simulink model "Simulink_ABS_Braking_Vehicle_Dynamics"  (R2024b)
settings: Solver=VariableStepAuto  StartTime=0.0  StopTime=10.0  RelTol=1e-3
values from neighbouring files (symbols this model uses):
  delta = 5 * pi/180    (= 0.0872664625997)    [ABS_MAtlab_Script_Automation.m]
  I_w = 1.12    [ABS_MAtlab_Script_Automation.m]
  lambda_bp = (0:0.05:1)'    [ABS_MAtlab_Script_Automation.m]
  m = 1400    [ABS_MAtlab_Script_Automation.m]
  mu_dry = ([0.00  0.40  0.80  0.97  1.00  0.98  0.96  0.94  0.92  0.90 0.88  0.85  0.83  0.81  0.79  0.77  0.75  0.73  0.72  0.71  0.70 ])'    [ABS_MAtlab_Script_Automation.m]
  mu_ice = ([0.00  0.05  0.10  0.12  0.13  0.14  0.14  0.14  0.14  0.14  0.14  0.14  0.14  0.14  0.14  0.14  0.14  0.14  0.14  0.14  0.14 ])'    [ABS_MAtlab_Script_Automation.m]
  mu_wet = ([0.00  0.25  0.45  0.55  0.60  0.62  0.61  0.60  0.59  0.58 0.57  0.56  0.55  0.54  0.53  0.52  0.50  0.48  0.46  0.44  0.42 ])'    [ABS_MAtlab_Script_Automation.m]
  r = 0.33    [ABS_MAtlab_Script_Automation.m]
  T_brake = 2000    [ABS_MAtlab_Script_Automation.m]
  v0 = 100/3.6    (= 27.7777777778)    [ABS_MAtlab_Script_Automation.m]
  w0 = v0/r    (= 84.1750841751)    [ABS_MAtlab_Script_Automation.m]
libraries: simulink x8, slpidlib x4
(part 1 of 2)
settings Model: Creator=mohammed omrez khan  LastModifiedBy=mohammed omrez khan

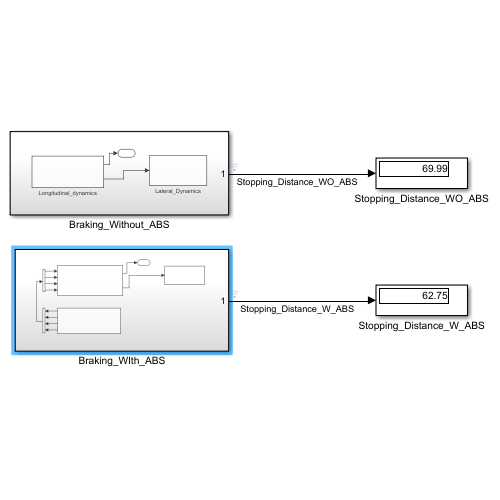
[thumbnail: Simulink's stored preview of the top-level diagram]
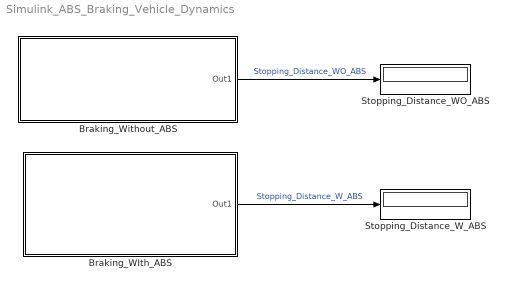
== system Simulink_ABS_Braking_Vehicle_Dynamics ==
  Braking_WIth_ABS : Subsystem
  Braking_Without_ABS : Subsystem
  Stopping_Distance_WO_ABS : Display
  Stopping_Distance_W_ABS : Display
  wires:
  Braking_Without_ABS/1(Out1) -> Stopping_Distance_WO_ABS/1  "Stopping_Distance_WO_ABS"
  Braking_WIth_ABS/1(Out1) -> Stopping_Distance_W_ABS/1  "Stopping_Distance_W_ABS"

== system Simulink_ABS_Braking_Vehicle_Dynamics/Braking_WIth_ABS ==
  Demux : Demux
  Lateral_Dynamics_ABS : Subsystem
  Longitudinal_Dynamics_ABS : Subsystem
  Mux : Mux
  Usage_ECS_Monitoring : Subsystem
      settings: PortSchema="{\"entries\":[{\"content\":{\"sides\":[{\"content\":{\"connectorIds\":[\"Out1\",\"Out2\",\"Out3\",\"Out4\"]},\"type\":\"ConnectorPlacement.EquallySpacedRectSide\",\"uuid\":\"f2e56514-8109-4cf8-b4cd-59c3b61fcd4b\"},{\"content\":{\"side\":\"RIGHT\"},\"type\":\"ConnectorPlacement.EquallySpacedRectSide\",\"uuid\":\"6eb04186-cc68-428c-910d-d8e45f75c5ef\"},{\"content\":{\"side\":\"TOP\"},\"type\":\"ConnectorPlacement.EquallySpacedRectSide\",\"uuid\":\"72babd61-98dc-4993-babf-b2ef769bf457\"}]},\"type\":\"ConnectorPlacement.EquallySpacedConnector\",\"uuid\":\"fac04954-b134-470d-b15d-7da1141ea9e2\"}],\"packageUris\":[\"http://schema.mathworks.com/mf0/Connector/R2020b\"],\"version\":\"1.0\"}"
  Out1 : Outport
  wires:
  Longitudinal_Dynamics_ABS/1(Out1) -> Out1/1
  Longitudinal_Dynamics_ABS/2(V_x) -> Lateral_Dynamics_ABS/1(V_x)
  Usage_ECS_Monitoring/1(Out1) -> Mux/1
  Usage_ECS_Monitoring/2(Out2) -> Mux/2
  Usage_ECS_Monitoring/3(Out3) -> Mux/3
  Usage_ECS_Monitoring/4(Out4) -> Mux/4
  Mux/1 -> Demux/1
  Demux/1 -> Longitudinal_Dynamics_ABS/1(In1)
  Demux/2 -> Longitudinal_Dynamics_ABS/2(In2)
  Demux/3 -> Longitudinal_Dynamics_ABS/3(In3)
  Demux/4 -> Longitudinal_Dynamics_ABS/4(In4)

== system Simulink_ABS_Braking_Vehicle_Dynamics/Braking_Without_ABS ==
  Lateral_Dynamics : Subsystem
  Longitudinal_dynamics : Subsystem
  Out1 : Outport
  wires:
  Longitudinal_dynamics/1(Out1) -> Out1/1
  Longitudinal_dynamics/2(V_x) -> Lateral_Dynamics/1(V_x)

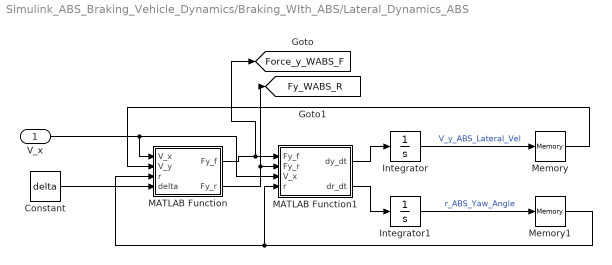
== system Simulink_ABS_Braking_Vehicle_Dynamics/Braking_WIth_ABS/Lateral_Dynamics_ABS ==
  V_x : Inport
  Constant : Constant  Value=delta
  Integrator : Integrator
  Integrator1 : Integrator
  MATLAB Function : MATLAB Function  TreatAsAtomicUnit=on
  MATLAB Function1 : MATLAB Function  TreatAsAtomicUnit=on
  Memory : Memory
  Memory1 : Memory
  tag scope: Force_y_WABS_F=global, Fy_WABS_R=global
  wires:
  MATLAB Function1/1(dy_dt) -> Integrator/1
  Constant/1 -> MATLAB Function/4(delta)
  MATLAB Function1/2(dr_dt) -> Integrator1/1
  MATLAB Function/1(Fy_f) -> [Force_y_WABS_F], MATLAB Function1/1(Fy_f)
  V_x/1 -> MATLAB Function/1(V_x), MATLAB Function1/3(V_x)
  Integrator/1 -> Memory/1  "V_y_ABS_Lateral_Vel"
  Memory/1 -> MATLAB Function/2(V_y)
  Integrator1/1 -> Memory1/1  "r_ABS_Yaw_Angle"
  Memory1/1 -> MATLAB Function/3(r), MATLAB Function1/4(r)
  MATLAB Function/2(Fy_r) -> [Fy_WABS_R], MATLAB Function1/2(Fy_r)

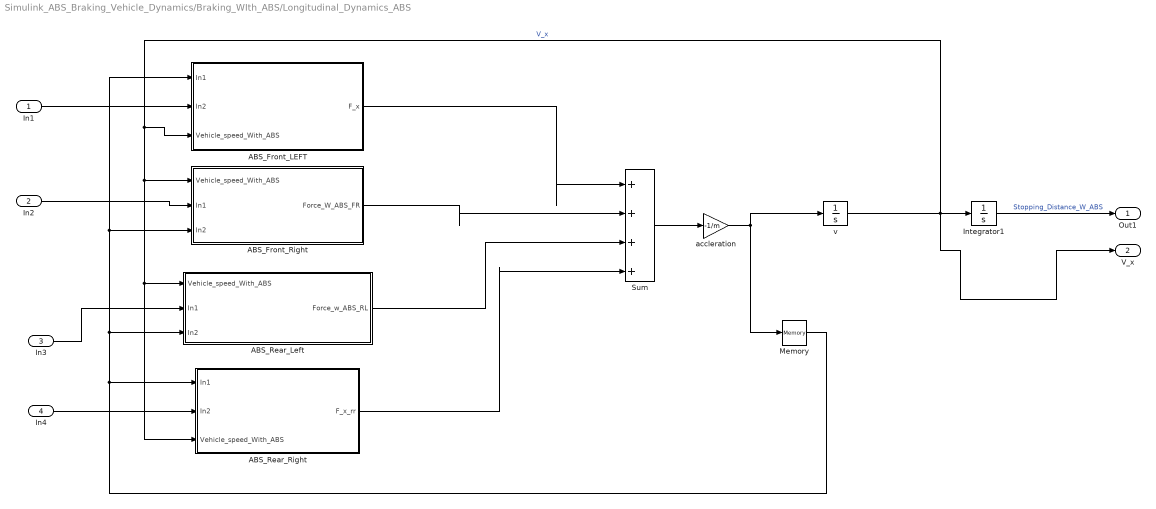
== system Simulink_ABS_Braking_Vehicle_Dynamics/Braking_WIth_ABS/Longitudinal_Dynamics_ABS ==
  In1 : Inport
  In2 : Inport  Port=2
  In3 : Inport  Port=3
  In4 : Inport  Port=4
  ABS_Front_LEFT : Subsystem
  ABS_Front_Right : Subsystem
  ABS_Rear_Left : Subsystem
  ABS_Rear_Right : Subsystem
  Integrator1 : Integrator
  Memory : Memory
  Sum : Sum  Inputs=|++++
  accleration : Gain  Gain=-1/m
  v : Integrator  InitialCondition=v0  LimitOutput=on  LowerSaturationLimit=0
  Out1 : Outport
  V_x : Outport  Port=2
  wires:
  Sum/1 -> accleration/1
  Memory/1 -> ABS_Front_LEFT/1(In1), ABS_Front_Right/3(In2), ABS_Rear_Left/3(In2), ABS_Rear_Right/1(In1)
  v/1 -> V_x/1, ABS_Rear_Right/3(Vehicle_speed_With_ABS), ABS_Rear_Left/1(Vehicle_speed_With_ABS), ABS_Front_Right/1(Vehicle_speed_With_ABS), ABS_Front_LEFT/3(Vehicle_speed_With_ABS), Integrator1/1  "V_x"
  accleration/1 -> v/1, Memory/1
  ABS_Rear_Right/1(F_x_rr) -> Sum/4
  ABS_Rear_Left/1(Force_w_ABS_RL) -> Sum/3
  ABS_Front_Right/1(Force_W_ABS_FR) -> Sum/2
  ABS_Front_LEFT/1(F_x) -> Sum/1
  Integrator1/1 -> Out1/1  "Stopping_Distance_W_ABS"
  In1/1 -> ABS_Front_LEFT/2(In2)
  In2/1 -> ABS_Front_Right/2(In1)
  In3/1 -> ABS_Rear_Left/2(In1)
  In4/1 -> ABS_Rear_Right/2(In2)

== system Simulink_ABS_Braking_Vehicle_Dynamics/Braking_WIth_ABS/Usage_ECS_Monitoring ==
  Front_Left Wheel : Subsystem
  Front_Right_Wheel : Subsystem
  Rear_Left_Wheel : Subsystem
  Rear_Right_Wheel : Subsystem
  Out1 : Outport
  Out2 : Outport  Port=2
  Out3 : Outport  Port=3
  Out4 : Outport  Port=4
  wires:
  Front_Left Wheel/1(Out1) -> Out1/1
  Front_Right_Wheel/1(Out1) -> Out2/1
  Rear_Left_Wheel/1(Out3) -> Out3/1
  Rear_Right_Wheel/1(Out3) -> Out4/1

== system Simulink_ABS_Braking_Vehicle_Dynamics/Braking_Without_ABS/Lateral_Dynamics ==
  V_x : Inport
  Constant : Constant  Value=delta
  Integrator : Integrator
  Integrator1 : Integrator
  MATLAB Function : MATLAB Function  TreatAsAtomicUnit=on
  MATLAB Function1 : MATLAB Function  TreatAsAtomicUnit=on
  Memory : Memory
  Memory1 : Memory
  wires:
  MATLAB Function/2(Fy_r) -> MATLAB Function1/2(Fy_r)
  MATLAB Function1/1(dy_dt) -> Integrator/1
  Constant/1 -> MATLAB Function/4(delta)
  MATLAB Function1/2(dr_dt) -> Integrator1/1
  MATLAB Function/1(Fy_f) -> MATLAB Function1/1(Fy_f)
  V_x/1 -> MATLAB Function/1(V_x), MATLAB Function1/3(V_x)
  Integrator/1 -> Memory/1  "V_y_velocity in Lateral"
  Memory/1 -> MATLAB Function/2(V_y)
  Integrator1/1 -> Memory1/1  "r_Yaw_Angle"
  Memory1/1 -> MATLAB Function1/4(r), MATLAB Function/3(r)

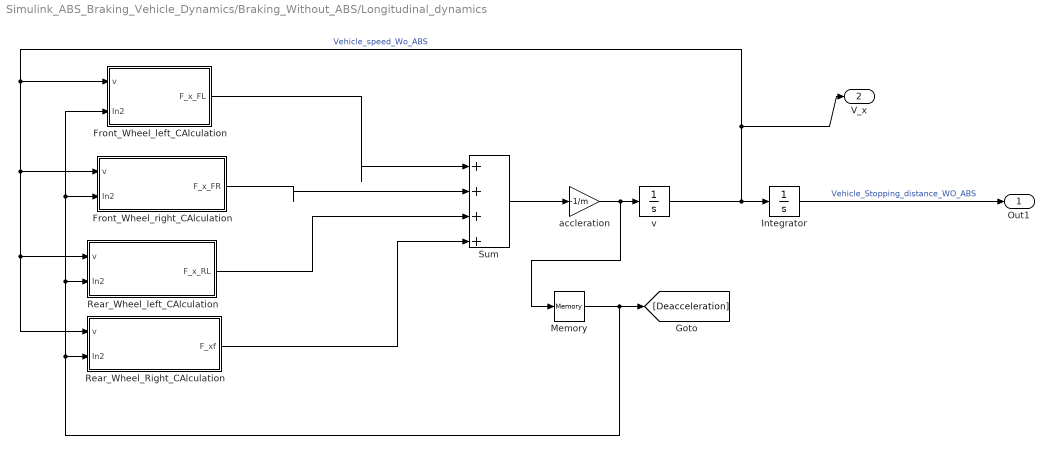
== system Simulink_ABS_Braking_Vehicle_Dynamics/Braking_Without_ABS/Longitudinal_dynamics ==
  Front_Wheel_left_CAlculation : Subsystem
  Front_Wheel_right_CAlculation : Subsystem
  Integrator : Integrator
  Memory : Memory
  Rear_Wheel_Right_CAlculation : Subsystem
  Rear_Wheel_left_CAlculation : Subsystem
  Sum : Sum  Inputs=|++++
  accleration : Gain  Gain=-1/m
  v : Integrator  InitialCondition=v0  LimitOutput=on  LowerSaturationLimit=0
  Out1 : Outport
  V_x : Outport  Port=2
  wires:
  Memory/1 -> Front_Wheel_left_CAlculation/2(In2), Front_Wheel_right_CAlculation/2(In2), Rear_Wheel_left_CAlculation/2(In2), Rear_Wheel_Right_CAlculation/2(In2), [Deacceleration]
  Front_Wheel_left_CAlculation/1(F_x_FL) -> Sum/1
  accleration/1 -> Memory/1, v/1
  Rear_Wheel_Right_CAlculation/1(F_xf) -> Sum/4
  Front_Wheel_right_CAlculation/1(F_x_FR) -> Sum/2
  v/1 -> Integrator/1, V_x/1, Rear_Wheel_Right_CAlculation/1(v), Rear_Wheel_left_CAlculation/1(v), Front_Wheel_right_CAlculation/1(v), Front_Wheel_left_CAlculation/1(v)  "Vehicle_speed_Wo_ABS"
  Sum/1 -> accleration/1
  Rear_Wheel_left_CAlculation/1(F_x_RL) -> Sum/3
  Integrator/1 -> Out1/1  "Vehicle_Stopping_distance_WO_ABS"

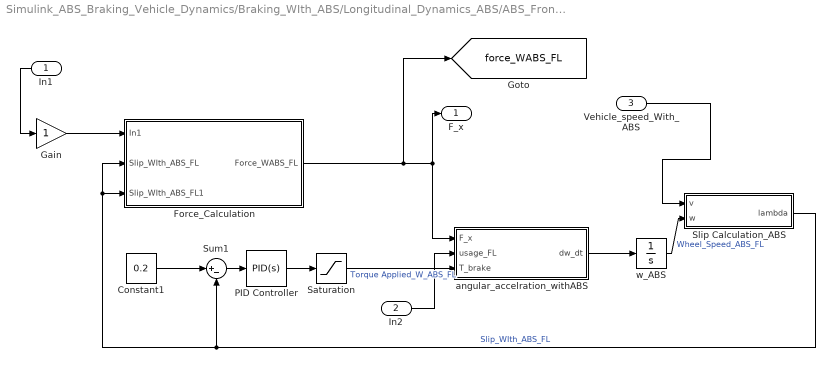
== system Simulink_ABS_Braking_Vehicle_Dynamics/Braking_WIth_ABS/Longitudinal_Dynamics_ABS/ABS_Front_LEFT ==
  In1 : Inport
  In2 : Inport  Port=2
  Vehicle_speed_With_ABS : Inport  Port=3
  Constant1 : Constant  Value=0.2
  Force_Calculation : Subsystem
  Gain : Gain
  PID Controller : slpidlib/PID Controller  Controller=PID  Form=Parallel  TimeDomain=Continuous-time  UseExternalTs=off  SampleTime=-1  IntegratorMethod=Forward Euler  FilterMethod=Forward Euler  ControllerParametersSource=internal  P=500000  I=500  UseKiTs=off  D=400  UseExternalDerivativeSource=off  N=100  UseFilter=on  TunerSelectOption=Transfer Function Based (PID Tuner App)  InitialConditionSource=internal  InitialConditionForIntegrator=0  InitialConditionForFilter=0  DifferentiatorICPrevScaledInput=0  ExternalReset=none  TrackingMode=off  Kt=1  LimitOutput=off  SatLimitsSource=internal  UpperSaturationLimit=inf  LowerSaturationLimit=-inf  LinearizeAsGain=on  AntiWindupMode=none  Kb=1  LimitIntegrator=off  UpperIntegratorSaturationLimit=inf  LowerIntegratorSaturationLimit=-inf  POutMin=[]  POutMax=[]  IOutMin=[]  IOutMax=[]  DOutMin=[]  DOutMax=[]  NOutMin=[]  NOutMax=[]  SumOutMin=[]  SumOutMax=[]  SaturationOutMin=[]  SaturationOutMax=[]  PParamMin=[]  PParamMax=[]  IParamMin=[]  IParamMax=[]  DParamMin=[]  DParamMax=[]  NParamMin=[]  NParamMax=[]  KbParamMin=[]  KbParamMax=[]  KtParamMin=[]  KtParamMax=[]  KbOutMin=[]  KbOutMax=[]  KtOutMin=[]  KtOutMax=[]  IntegratorOutMin=[]  IntegratorOutMax=[]  FilterOutMin=[]  FilterOutMax=[]  SumI1OutMin=[]  SumI1OutMax=[]  SumI2OutMin=[]  SumI2OutMax=[]  SumI3OutMin=[]  SumI3OutMax=[]  SumI4OutMin=[]  SumI4OutMax=[]  SumDOutMin=[]  SumDOutMax=[]  DifferentiatorOutMin=[]  DifferentiatorOutMax=[]  FilterDiffOutCoefMin=[]  FilterDiffOutCoefMax=[]  ReciprocalOutMin=[]  ReciprocalOutMax=[]  SumDenOutMin=[]  SumDenOutMax=[]  SumNumOutMin=[]  SumNumOutMax=[]  DivideOutMin=[]  DivideOutMax=[]  UdiffTsProdOutMin=[]  UdiffTsProdOutMax=[]  NTsProdOutMin=[]  NTsProdOutMax=[]  UintegralTsProdOutMin=[]  UintegralTsProdOutMax=[]  UngainTsProdOutMin=[]  UngainTsProdOutMax=[]  ClampingZeroOutDataTypeStr=Inherit: Inherit via back propagation  ClampingZeroOutMin=[]  ClampingZeroOutMax=[]  FilterDenConstantOutDataTypeStr=Inherit: Inherit via back propagation  FilterDenConstantOutMin=[]  FilterDenConstantOutMax=[]  PCopyOutDataTypeStr=Inherit: Inherit via back propagation  PCopyOutMin=[]  PCopyOutMax=[]  NCopyOutDataTypeStr=Inherit: Inherit via back propagation  NCopyOutMin=[]  NCopyOutMax=[]  IntegratorContinuousStateAttributes=''  IntegratorStateMustResolveToSignalObject=off  IntegratorRTWStateStorageClass=Auto  FilterContinuousStateAttributes=''  FilterStateMustResolveToSignalObject=off  FilterRTWStateStorageClass=Auto  ParallelPVariant=InternalParameters  IdealPVariant=Disabled  IVariant=InternalParameters  DVariant=InternalParameters  IntegratorVariant=Continuous  SatVariant=Disabled  AWVariant=Passthrough  PCopyVariant=Disabled  TRVariant=Disabled  FdbkBlocksVariant=Forward  IdealPFdbkVariant=Disabled  SatFdbkVariant=Disabled  DerivativeFilterVariant=ContFilter  NVariant=InternalParameters  NCopyVariant=Disabled  FilterICVariant=InternalICsFilter  IntegratorICVariant=InternalICs  ExternalResetVariant=Disabled  TRSumVariant=Passthrough  SumFdbkVariant=Disabled  SumVariant=Sum_PID  TsampFilterVariant=InternalTs  TsampNgainVariant=Passthrough  TsampIntegralVariant=Disabled_SignalSpec  ExternalSaturationOutDataTypeStr=Inherit: Same as second input  DerivativeSourceVariant=ErrorSignal  PreIntVariant=InternalPreInt
  Saturation : Saturate  UpperLimit=2000  LowerLimit=0
  Slip Calculation_ABS : Subsystem
  Sum1 : Sum  Inputs=|+-
  angular_accelration_withABS : Subsystem
  w_ABS : Integrator  InitialCondition=w0  LimitOutput=on  LowerSaturationLimit=0
  F_x : Outport
  tag scope: force_WABS_FL=global
  wires:
  Sum1/1 -> PID Controller/1
  angular_accelration_withABS/1(dw_dt) -> w_ABS/1
  Force_Calculation/1(Force_WABS_FL) -> angular_accelration_withABS/1(F_x), F_x/1, [force_WABS_FL]
  Slip Calculation_ABS/1(lambda) -> Force_Calculation/2(Slip_WIth_ABS_FL), Force_Calculation/3(Slip_WIth_ABS_FL1), Sum1/2  "Slip_WIth_ABS_FL"
  PID Controller/1 -> Saturation/1
  Gain/1 -> Force_Calculation/1(In1)
  w_ABS/1 -> Slip Calculation_ABS/2(w)  "Wheel_Speed_ABS_FL"
  Constant1/1 -> Sum1/1
  In1/1 -> Gain/1
  Vehicle_speed_With_ABS/1 -> Slip Calculation_ABS/1(v)
  Saturation/1 -> angular_accelration_withABS/3(T_brake)  "Torque Applied_W_ABS_FL"
  In2/1 -> angular_accelration_withABS/2(usage_FL)

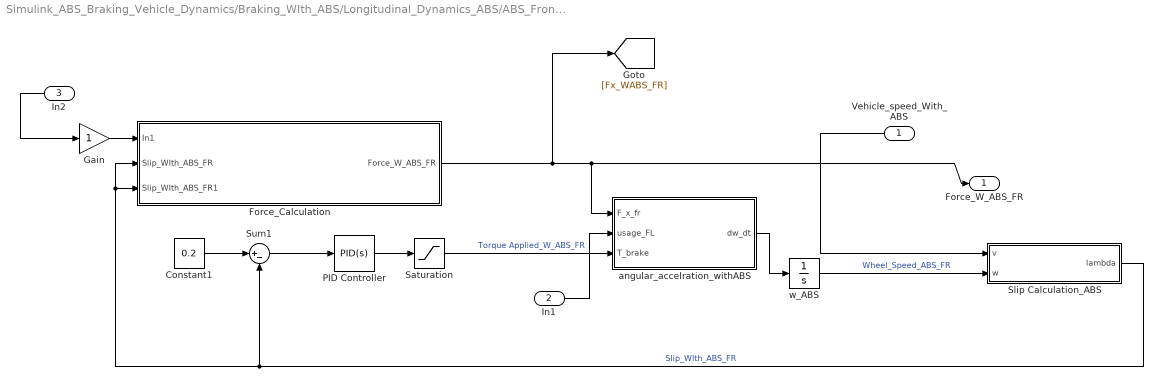
== system Simulink_ABS_Braking_Vehicle_Dynamics/Braking_WIth_ABS/Longitudinal_Dynamics_ABS/ABS_Front_Right ==
  Vehicle_speed_With_ABS : Inport
  In1 : Inport  Port=2
  In2 : Inport  Port=3
  Constant1 : Constant  Value=0.2
  Force_Calculation : Subsystem
  Gain : Gain
  PID Controller : slpidlib/PID Controller  Controller=PID  Form=Parallel  TimeDomain=Continuous-time  UseExternalTs=off  SampleTime=-1  IntegratorMethod=Forward Euler  FilterMethod=Forward Euler  ControllerParametersSource=internal  P=500000  I=500  UseKiTs=off  D=400  UseExternalDerivativeSource=off  N=100  UseFilter=on  TunerSelectOption=Transfer Function Based (PID Tuner App)  InitialConditionSource=internal  InitialConditionForIntegrator=0  InitialConditionForFilter=0  DifferentiatorICPrevScaledInput=0  ExternalReset=none  TrackingMode=off  Kt=1  LimitOutput=off  SatLimitsSource=internal  UpperSaturationLimit=inf  LowerSaturationLimit=-inf  LinearizeAsGain=on  AntiWindupMode=none  Kb=1  LimitIntegrator=off  UpperIntegratorSaturationLimit=inf  LowerIntegratorSaturationLimit=-inf  POutMin=[]  POutMax=[]  IOutMin=[]  IOutMax=[]  DOutMin=[]  DOutMax=[]  NOutMin=[]  NOutMax=[]  SumOutMin=[]  SumOutMax=[]  SaturationOutMin=[]  SaturationOutMax=[]  PParamMin=[]  PParamMax=[]  IParamMin=[]  IParamMax=[]  DParamMin=[]  DParamMax=[]  NParamMin=[]  NParamMax=[]  KbParamMin=[]  KbParamMax=[]  KtParamMin=[]  KtParamMax=[]  KbOutMin=[]  KbOutMax=[]  KtOutMin=[]  KtOutMax=[]  IntegratorOutMin=[]  IntegratorOutMax=[]  FilterOutMin=[]  FilterOutMax=[]  SumI1OutMin=[]  SumI1OutMax=[]  SumI2OutMin=[]  SumI2OutMax=[]  SumI3OutMin=[]  SumI3OutMax=[]  SumI4OutMin=[]  SumI4OutMax=[]  SumDOutMin=[]  SumDOutMax=[]  DifferentiatorOutMin=[]  DifferentiatorOutMax=[]  FilterDiffOutCoefMin=[]  FilterDiffOutCoefMax=[]  ReciprocalOutMin=[]  ReciprocalOutMax=[]  SumDenOutMin=[]  SumDenOutMax=[]  SumNumOutMin=[]  SumNumOutMax=[]  DivideOutMin=[]  DivideOutMax=[]  UdiffTsProdOutMin=[]  UdiffTsProdOutMax=[]  NTsProdOutMin=[]  NTsProdOutMax=[]  UintegralTsProdOutMin=[]  UintegralTsProdOutMax=[]  UngainTsProdOutMin=[]  UngainTsProdOutMax=[]  ClampingZeroOutDataTypeStr=Inherit: Inherit via back propagation  ClampingZeroOutMin=[]  ClampingZeroOutMax=[]  FilterDenConstantOutDataTypeStr=Inherit: Inherit via back propagation  FilterDenConstantOutMin=[]  FilterDenConstantOutMax=[]  PCopyOutDataTypeStr=Inherit: Inherit via back propagation  PCopyOutMin=[]  PCopyOutMax=[]  NCopyOutDataTypeStr=Inherit: Inherit via back propagation  NCopyOutMin=[]  NCopyOutMax=[]  IntegratorContinuousStateAttributes=''  IntegratorStateMustResolveToSignalObject=off  IntegratorRTWStateStorageClass=Auto  FilterContinuousStateAttributes=''  FilterStateMustResolveToSignalObject=off  FilterRTWStateStorageClass=Auto  ParallelPVariant=InternalParameters  IdealPVariant=Disabled  IVariant=InternalParameters  DVariant=InternalParameters  IntegratorVariant=Continuous  SatVariant=Disabled  AWVariant=Passthrough  PCopyVariant=Disabled  TRVariant=Disabled  FdbkBlocksVariant=Forward  IdealPFdbkVariant=Disabled  SatFdbkVariant=Disabled  DerivativeFilterVariant=ContFilter  NVariant=InternalParameters  NCopyVariant=Disabled  FilterICVariant=InternalICsFilter  IntegratorICVariant=InternalICs  ExternalResetVariant=Disabled  TRSumVariant=Passthrough  SumFdbkVariant=Disabled  SumVariant=Sum_PID  TsampFilterVariant=InternalTs  TsampNgainVariant=Passthrough  TsampIntegralVariant=Disabled_SignalSpec  ExternalSaturationOutDataTypeStr=Inherit: Same as second input  DerivativeSourceVariant=ErrorSignal  PreIntVariant=InternalPreInt
  Saturation : Saturate  UpperLimit=2000  LowerLimit=0
  Slip Calculation_ABS : Subsystem
  Sum1 : Sum  Inputs=|+-
  angular_accelration_withABS : Subsystem
  w_ABS : Integrator  InitialCondition=w0  LimitOutput=on  LowerSaturationLimit=0
  Force_W_ABS_FR : Outport
  wires:
  w_ABS/1 -> Slip Calculation_ABS/2(w)  "Wheel_Speed_ABS_FR"
  Force_Calculation/1(Force_W_ABS_FR) -> [Fx_WABS_FR], angular_accelration_withABS/1(F_x_fr), Force_W_ABS_FR/1
  Gain/1 -> Force_Calculation/1(In1)
  PID Controller/1 -> Saturation/1
  angular_accelration_withABS/1(dw_dt) -> w_ABS/1
  Sum1/1 -> PID Controller/1
  Constant1/1 -> Sum1/1
  Slip Calculation_ABS/1(lambda) -> Force_Calculation/2(Slip_WIth_ABS_FR), Force_Calculation/3(Slip_WIth_ABS_FR1), Sum1/2  "Slip_WIth_ABS_FR"
  In2/1 -> Gain/1
  Vehicle_speed_With_ABS/1 -> Slip Calculation_ABS/1(v)
  Saturation/1 -> angular_accelration_withABS/3(T_brake)  "Torque Applied_W_ABS_FR"
  In1/1 -> angular_accelration_withABS/2(usage_FL)

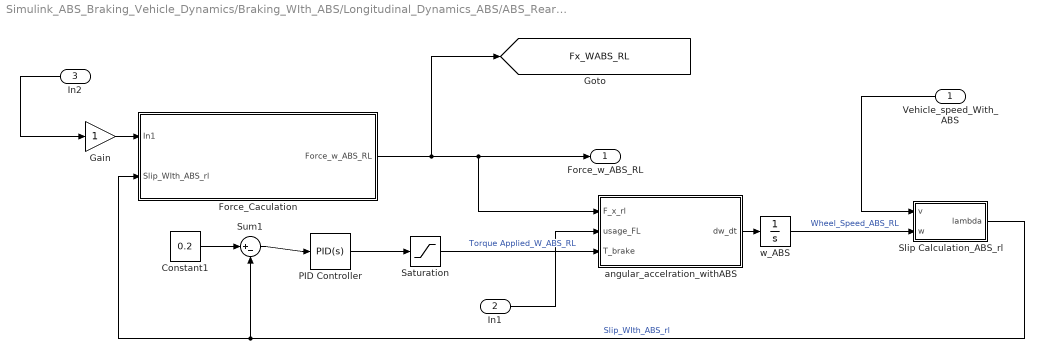
== system Simulink_ABS_Braking_Vehicle_Dynamics/Braking_WIth_ABS/Longitudinal_Dynamics_ABS/ABS_Rear_Left ==
  Vehicle_speed_With_ABS : Inport
  In1 : Inport  Port=2
  In2 : Inport  Port=3
  Constant1 : Constant  Value=0.2
  Force_Caculation : Subsystem
  Gain : Gain
  PID Controller : slpidlib/PID Controller  Controller=PID  Form=Parallel  TimeDomain=Continuous-time  UseExternalTs=off  SampleTime=-1  IntegratorMethod=Forward Euler  FilterMethod=Forward Euler  ControllerParametersSource=internal  P=500000  I=500  UseKiTs=off  D=400  UseExternalDerivativeSource=off  N=100  UseFilter=on  TunerSelectOption=Transfer Function Based (PID Tuner App)  InitialConditionSource=internal  InitialConditionForIntegrator=0  InitialConditionForFilter=0  DifferentiatorICPrevScaledInput=0  ExternalReset=none  TrackingMode=off  Kt=1  LimitOutput=off  SatLimitsSource=internal  UpperSaturationLimit=inf  LowerSaturationLimit=-inf  LinearizeAsGain=on  AntiWindupMode=none  Kb=1  LimitIntegrator=off  UpperIntegratorSaturationLimit=inf  LowerIntegratorSaturationLimit=-inf  POutMin=[]  POutMax=[]  IOutMin=[]  IOutMax=[]  DOutMin=[]  DOutMax=[]  NOutMin=[]  NOutMax=[]  SumOutMin=[]  SumOutMax=[]  SaturationOutMin=[]  SaturationOutMax=[]  PParamMin=[]  PParamMax=[]  IParamMin=[]  IParamMax=[]  DParamMin=[]  DParamMax=[]  NParamMin=[]  NParamMax=[]  KbParamMin=[]  KbParamMax=[]  KtParamMin=[]  KtParamMax=[]  KbOutMin=[]  KbOutMax=[]  KtOutMin=[]  KtOutMax=[]  IntegratorOutMin=[]  IntegratorOutMax=[]  FilterOutMin=[]  FilterOutMax=[]  SumI1OutMin=[]  SumI1OutMax=[]  SumI2OutMin=[]  SumI2OutMax=[]  SumI3OutMin=[]  SumI3OutMax=[]  SumI4OutMin=[]  SumI4OutMax=[]  SumDOutMin=[]  SumDOutMax=[]  DifferentiatorOutMin=[]  DifferentiatorOutMax=[]  FilterDiffOutCoefMin=[]  FilterDiffOutCoefMax=[]  ReciprocalOutMin=[]  ReciprocalOutMax=[]  SumDenOutMin=[]  SumDenOutMax=[]  SumNumOutMin=[]  SumNumOutMax=[]  DivideOutMin=[]  DivideOutMax=[]  UdiffTsProdOutMin=[]  UdiffTsProdOutMax=[]  NTsProdOutMin=[]  NTsProdOutMax=[]  UintegralTsProdOutMin=[]  UintegralTsProdOutMax=[]  UngainTsProdOutMin=[]  UngainTsProdOutMax=[]  ClampingZeroOutDataTypeStr=Inherit: Inherit via back propagation  ClampingZeroOutMin=[]  ClampingZeroOutMax=[]  FilterDenConstantOutDataTypeStr=Inherit: Inherit via back propagation  FilterDenConstantOutMin=[]  FilterDenConstantOutMax=[]  PCopyOutDataTypeStr=Inherit: Inherit via back propagation  PCopyOutMin=[]  PCopyOutMax=[]  NCopyOutDataTypeStr=Inherit: Inherit via back propagation  NCopyOutMin=[]  NCopyOutMax=[]  IntegratorContinuousStateAttributes=''  IntegratorStateMustResolveToSignalObject=off  IntegratorRTWStateStorageClass=Auto  FilterContinuousStateAttributes=''  FilterStateMustResolveToSignalObject=off  FilterRTWStateStorageClass=Auto  ParallelPVariant=InternalParameters  IdealPVariant=Disabled  IVariant=InternalParameters  DVariant=InternalParameters  IntegratorVariant=Continuous  SatVariant=Disabled  AWVariant=Passthrough  PCopyVariant=Disabled  TRVariant=Disabled  FdbkBlocksVariant=Forward  IdealPFdbkVariant=Disabled  SatFdbkVariant=Disabled  DerivativeFilterVariant=ContFilter  NVariant=InternalParameters  NCopyVariant=Disabled  FilterICVariant=InternalICsFilter  IntegratorICVariant=InternalICs  ExternalResetVariant=Disabled  TRSumVariant=Passthrough  SumFdbkVariant=Disabled  SumVariant=Sum_PID  TsampFilterVariant=InternalTs  TsampNgainVariant=Passthrough  TsampIntegralVariant=Disabled_SignalSpec  ExternalSaturationOutDataTypeStr=Inherit: Same as second input  DerivativeSourceVariant=ErrorSignal  PreIntVariant=InternalPreInt
  Saturation : Saturate  UpperLimit=2000  LowerLimit=0
  Slip Calculation_ABS_rl : Subsystem
  Sum1 : Sum  Inputs=|+-
  angular_accelration_withABS : Subsystem
  w_ABS : Integrator  InitialCondition=w0  LimitOutput=on  LowerSaturationLimit=0
  Force_w_ABS_RL : Outport
  tag scope: Fx_WABS_RL=global
  wires:
  Sum1/1 -> PID Controller/1
  Vehicle_speed_With_ABS/1 -> Slip Calculation_ABS_rl/1(v)
  Slip Calculation_ABS_rl/1(lambda) -> Force_Caculation/2(Slip_WIth_ABS_rl), Sum1/2  "Slip_WIth_ABS_rl"
  PID Controller/1 -> Saturation/1
  Constant1/1 -> Sum1/1
  angular_accelration_withABS/1(dw_dt) -> w_ABS/1
  w_ABS/1 -> Slip Calculation_ABS_rl/2(w)  "Wheel_Speed_ABS_RL"
  In2/1 -> Gain/1
  Gain/1 -> Force_Caculation/1(In1)
  Saturation/1 -> angular_accelration_withABS/3(T_brake)  "Torque Applied_W_ABS_RL"
  Force_Caculation/1(Force_w_ABS_RL) -> [Fx_WABS_RL], angular_accelration_withABS/1(F_x_rl), Force_w_ABS_RL/1
  In1/1 -> angular_accelration_withABS/2(usage_FL)

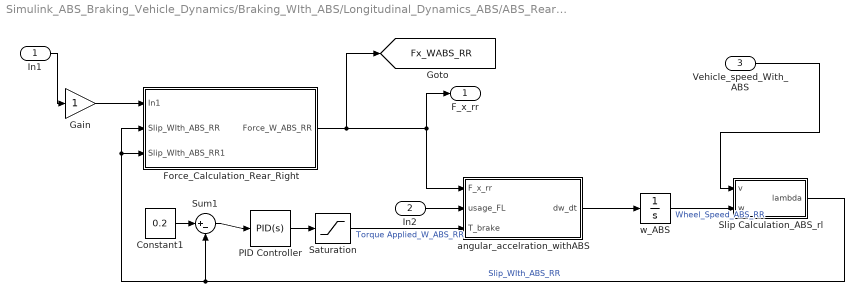
== system Simulink_ABS_Braking_Vehicle_Dynamics/Braking_WIth_ABS/Longitudinal_Dynamics_ABS/ABS_Rear_Right ==
  In1 : Inport
  In2 : Inport  Port=2
  Vehicle_speed_With_ABS : Inport  Port=3
  Constant1 : Constant  Value=0.2
  Force_Calculation_Rear_Right : Subsystem
  Gain : Gain
  PID Controller : slpidlib/PID Controller  Controller=PID  Form=Parallel  TimeDomain=Continuous-time  UseExternalTs=off  SampleTime=-1  IntegratorMethod=Forward Euler  FilterMethod=Forward Euler  ControllerParametersSource=internal  P=500000  I=500  UseKiTs=off  D=400  UseExternalDerivativeSource=off  N=100  UseFilter=on  TunerSelectOption=Transfer Function Based (PID Tuner App)  InitialConditionSource=internal  InitialConditionForIntegrator=0  InitialConditionForFilter=0  DifferentiatorICPrevScaledInput=0  ExternalReset=none  TrackingMode=off  Kt=1  LimitOutput=off  SatLimitsSource=internal  UpperSaturationLimit=inf  LowerSaturationLimit=-inf  LinearizeAsGain=on  AntiWindupMode=none  Kb=1  LimitIntegrator=off  UpperIntegratorSaturationLimit=inf  LowerIntegratorSaturationLimit=-inf  POutMin=[]  POutMax=[]  IOutMin=[]  IOutMax=[]  DOutMin=[]  DOutMax=[]  NOutMin=[]  NOutMax=[]  SumOutMin=[]  SumOutMax=[]  SaturationOutMin=[]  SaturationOutMax=[]  PParamMin=[]  PParamMax=[]  IParamMin=[]  IParamMax=[]  DParamMin=[]  DParamMax=[]  NParamMin=[]  NParamMax=[]  KbParamMin=[]  KbParamMax=[]  KtParamMin=[]  KtParamMax=[]  KbOutMin=[]  KbOutMax=[]  KtOutMin=[]  KtOutMax=[]  IntegratorOutMin=[]  IntegratorOutMax=[]  FilterOutMin=[]  FilterOutMax=[]  SumI1OutMin=[]  SumI1OutMax=[]  SumI2OutMin=[]  SumI2OutMax=[]  SumI3OutMin=[]  SumI3OutMax=[]  SumI4OutMin=[]  SumI4OutMax=[]  SumDOutMin=[]  SumDOutMax=[]  DifferentiatorOutMin=[]  DifferentiatorOutMax=[]  FilterDiffOutCoefMin=[]  FilterDiffOutCoefMax=[]  ReciprocalOutMin=[]  ReciprocalOutMax=[]  SumDenOutMin=[]  SumDenOutMax=[]  SumNumOutMin=[]  SumNumOutMax=[]  DivideOutMin=[]  DivideOutMax=[]  UdiffTsProdOutMin=[]  UdiffTsProdOutMax=[]  NTsProdOutMin=[]  NTsProdOutMax=[]  UintegralTsProdOutMin=[]  UintegralTsProdOutMax=[]  UngainTsProdOutMin=[]  UngainTsProdOutMax=[]  ClampingZeroOutDataTypeStr=Inherit: Inherit via back propagation  ClampingZeroOutMin=[]  ClampingZeroOutMax=[]  FilterDenConstantOutDataTypeStr=Inherit: Inherit via back propagation  FilterDenConstantOutMin=[]  FilterDenConstantOutMax=[]  PCopyOutDataTypeStr=Inherit: Inherit via back propagation  PCopyOutMin=[]  PCopyOutMax=[]  NCopyOutDataTypeStr=Inherit: Inherit via back propagation  NCopyOutMin=[]  NCopyOutMax=[]  IntegratorContinuousStateAttributes=''  IntegratorStateMustResolveToSignalObject=off  IntegratorRTWStateStorageClass=Auto  FilterContinuousStateAttributes=''  FilterStateMustResolveToSignalObject=off  FilterRTWStateStorageClass=Auto  ParallelPVariant=InternalParameters  IdealPVariant=Disabled  IVariant=InternalParameters  DVariant=InternalParameters  IntegratorVariant=Continuous  SatVariant=Disabled  AWVariant=Passthrough  PCopyVariant=Disabled  TRVariant=Disabled  FdbkBlocksVariant=Forward  IdealPFdbkVariant=Disabled  SatFdbkVariant=Disabled  DerivativeFilterVariant=ContFilter  NVariant=InternalParameters  NCopyVariant=Disabled  FilterICVariant=InternalICsFilter  IntegratorICVariant=InternalICs  ExternalResetVariant=Disabled  TRSumVariant=Passthrough  SumFdbkVariant=Disabled  SumVariant=Sum_PID  TsampFilterVariant=InternalTs  TsampNgainVariant=Passthrough  TsampIntegralVariant=Disabled_SignalSpec  ExternalSaturationOutDataTypeStr=Inherit: Same as second input  DerivativeSourceVariant=ErrorSignal  PreIntVariant=InternalPreInt
  Saturation : Saturate  UpperLimit=2000  LowerLimit=0
  Slip Calculation_ABS_rl : Subsystem
  Sum1 : Sum  Inputs=|+-
  angular_accelration_withABS : Subsystem
  w_ABS : Integrator  InitialCondition=w0  LimitOutput=on  LowerSaturationLimit=0
  F_x_rr : Outport
  tag scope: Fx_WABS_RR=global
  wires:
  PID Controller/1 -> Saturation/1
  Slip Calculation_ABS_rl/1(lambda) -> Force_Calculation_Rear_Right/2(Slip_WIth_ABS_RR), Force_Calculation_Rear_Right/3(Slip_WIth_ABS_RR1), Sum1/2  "Slip_WIth_ABS_RR"
  angular_accelration_withABS/1(dw_dt) -> w_ABS/1
  Force_Calculation_Rear_Right/1(Force_W_ABS_RR) -> [Fx_WABS_RR], angular_accelration_withABS/1(F_x_rr), F_x_rr/1
  Gain/1 -> Force_Calculation_Rear_Right/1(In1)
  Constant1/1 -> Sum1/1
  Sum1/1 -> PID Controller/1
  Vehicle_speed_With_ABS/1 -> Slip Calculation_ABS_rl/1(v)
  In1/1 -> Gain/1
  w_ABS/1 -> Slip Calculation_ABS_rl/2(w)  "Wheel_Speed_ABS_RR"
  Saturation/1 -> angular_accelration_withABS/3(T_brake)  "Torque Applied_W_ABS_RR"
  In2/1 -> angular_accelration_withABS/2(usage_FL)

== system Simulink_ABS_Braking_Vehicle_Dynamics/Braking_WIth_ABS/Usage_ECS_Monitoring/Front_Left Wheel ==
  Gain : Gain  Gain=0.5
  MATLAB Function : MATLAB Function  TreatAsAtomicUnit=on
  Memory : Memory
  Scope : Scope
  Out1 : Outport
  wires:
  [Force_z_FL] -> MATLAB Function/3(Fz)
  MATLAB Function/1(usage_FL) -> [Usage_ABS_FL], Scope/1, Memory/1  "Usage_ABS_FL"
  Memory/1 -> Out1/1
  Gain/1 -> MATLAB Function/2(Fy)
  [Mu_WABS_FL] -> MATLAB Function/4(mu)
  [force_WABS_FL] -> MATLAB Function/1(Fx)
  [Force_y_WABS_F] -> Gain/1

== system Simulink_ABS_Braking_Vehicle_Dynamics/Braking_WIth_ABS/Usage_ECS_Monitoring/Front_Right_Wheel ==
  Gain : Gain  Gain=0.5
  MATLAB Function : MATLAB Function  TreatAsAtomicUnit=on
  Memory : Memory
  Scope : Scope
  Out1 : Outport
  wires:
  [Force_y_WABS_F] -> Gain/1
  [Fx_WABS_FR] -> MATLAB Function/1(Fx)
  [Mu_WABS_FR] -> MATLAB Function/4(mu)
  Gain/1 -> MATLAB Function/2(Fy)
  Memory/1 -> Out1/1
  MATLAB Function/1(usage_FL) -> [Usage_ABS_FL], Memory/1, Scope/1  "Usage_ABS_FR"
  [Fz_WABS_FR] -> MATLAB Function/3(Fz)

== system Simulink_ABS_Braking_Vehicle_Dynamics/Braking_WIth_ABS/Usage_ECS_Monitoring/Rear_Left_Wheel ==
  Gain : Gain  Gain=0.5
  MATLAB Function : MATLAB Function  TreatAsAtomicUnit=on
  Memory : Memory
  Scope : Scope
  Out3 : Outport
  wires:
  [Fz_WABS_RL] -> MATLAB Function/3(Fz)
  MATLAB Function/1(usage_FL) -> [Usage_ABS_FL], Scope/1, Memory/1  "USAGE_ABS_RL"
  Memory/1 -> Out3/1
  Gain/1 -> MATLAB Function/2(Fy)
  [Mu_WABS_RL] -> MATLAB Function/4(mu)
  [Fx_WABS_RL] -> MATLAB Function/1(Fx)
  [Fy_WABS_R] -> Gain/1

== system Simulink_ABS_Braking_Vehicle_Dynamics/Braking_WIth_ABS/Usage_ECS_Monitoring/Rear_Right_Wheel ==
  Gain : Gain  Gain=0.5
  MATLAB Function : MATLAB Function  TreatAsAtomicUnit=on
  Memory : Memory
  Scope : Scope
  Out3 : Outport
  wires:
  [Fy_WABS_R] -> Gain/1
  [Fx_WABS_RR] -> MATLAB Function/1(Fx)
  [Mu_WABS_RR] -> MATLAB Function/4(mu)
  Gain/1 -> MATLAB Function/2(Fy)
  Memory/1 -> Out3/1
  MATLAB Function/1(usage_FL) -> Memory/1, Scope/1, [Usage_ABS_RR]  "Usage_ABS_RR"
  [Fz_WABS_RR] -> MATLAB Function/3(Fz)

== system Simulink_ABS_Braking_Vehicle_Dynamics/Braking_Without_ABS/Longitudinal_dynamics/Front_Wheel_left_CAlculation ==
  v : Inport
  In2 : Inport  Port=2
  Scope : Scope
  Slip Calculation : Subsystem
  Vehicle Speed_Block : Subsystem
  angular_accelration_Wo_ABS : Subsystem
  w : Integrator  InitialCondition=w0  LimitOutput=on  LowerSaturationLimit=0
  F_x_FL : Outport
  wires:
  Vehicle Speed_Block/1(F_x) -> F_x_FL/1, angular_accelration_Wo_ABS/1(F_xf)
  w/1 -> Slip Calculation/2(w)  "Wheel_Speed_Wo_ABS_FL"
  Slip Calculation/1(lambda) -> Scope/1  "Slip_Wihout_ABS_FL"
  angular_accelration_Wo_ABS/1(dw_dt) -> w/1
  v/1 -> Slip Calculation/1(v)
  In2/1 -> Vehicle Speed_Block/1(a)

== system Simulink_ABS_Braking_Vehicle_Dynamics/Braking_Without_ABS/Longitudinal_dynamics/Front_Wheel_right_CAlculation ==
  v : Inport
  In2 : Inport  Port=2
  Scope : Scope
  Slip Calculation : Subsystem
  Vehicle Speed_Block : Subsystem
  angular_accelration_Wo_ABS : Subsystem
  w : Integrator  InitialCondition=w0  LimitOutput=on  LowerSaturationLimit=0
  F_x_FR : Outport
  wires:
  w/1 -> Slip Calculation/2(w)  "Wheel_Speed_Wo_ABS_FR"
  angular_accelration_Wo_ABS/1(dw_dt) -> w/1
  v/1 -> Slip Calculation/1(v)
  Vehicle Speed_Block/1(F_x_fr) -> angular_accelration_Wo_ABS/1(F_x_fr), F_x_FR/1
  Slip Calculation/1(lambda) -> Scope/1  "Slip_Wihout_ABS_FR"
  In2/1 -> Vehicle Speed_Block/1(a)

== system Simulink_ABS_Braking_Vehicle_Dynamics/Braking_Without_ABS/Longitudinal_dynamics/Rear_Wheel_Right_CAlculation ==
  v : Inport
  In2 : Inport  Port=2
  Scope : Scope
  Slip Calculation : Subsystem
  Vehicle Speed_Block : Subsystem
  angular_accelration_Wo_ABS : Subsystem
  w : Integrator  InitialCondition=w0  LimitOutput=on  LowerSaturationLimit=0
  F_xf : Outport
  wires:
  Slip Calculation/1(lambda) -> Scope/1  "Slip_Wihout_ABS_F1"
  Vehicle Speed_Block/1(F_x_RR) -> F_xf/1, angular_accelration_Wo_ABS/1(F_x_RR)
  angular_accelration_Wo_ABS/1(dw_dt) -> w/1
  w/1 -> Slip Calculation/2(w)  "Wheel_Speed_Wo_ABS_F"
  v/1 -> Slip Calculation/1(v)
  In2/1 -> Vehicle Speed_Block/1(a)

== system Simulink_ABS_Braking_Vehicle_Dynamics/Braking_Without_ABS/Longitudinal_dynamics/Rear_Wheel_left_CAlculation ==
  v : Inport
  In2 : Inport  Port=2
  Scope : Scope
  Slip Calculation : Subsystem
  Vehicle Speed_Block : Subsystem
  angular_accelration_Wo_ABS : Subsystem
  w : Integrator  InitialCondition=w0  LimitOutput=on  LowerSaturationLimit=0
  F_x_RL : Outport
  wires:
  Vehicle Speed_Block/1(F_x_RL) -> F_x_RL/1, angular_accelration_Wo_ABS/1(F_x_RL)
  Slip Calculation/1(lambda) -> Scope/1  "Slip_Wihout_ABS_RL"
  w/1 -> Slip Calculation/2(w)  "Wheel_Speed_Wo_ABS_RL"
  angular_accelration_Wo_ABS/1(dw_dt) -> w/1
  v/1 -> Slip Calculation/1(v)
  In2/1 -> Vehicle Speed_Block/1(a)

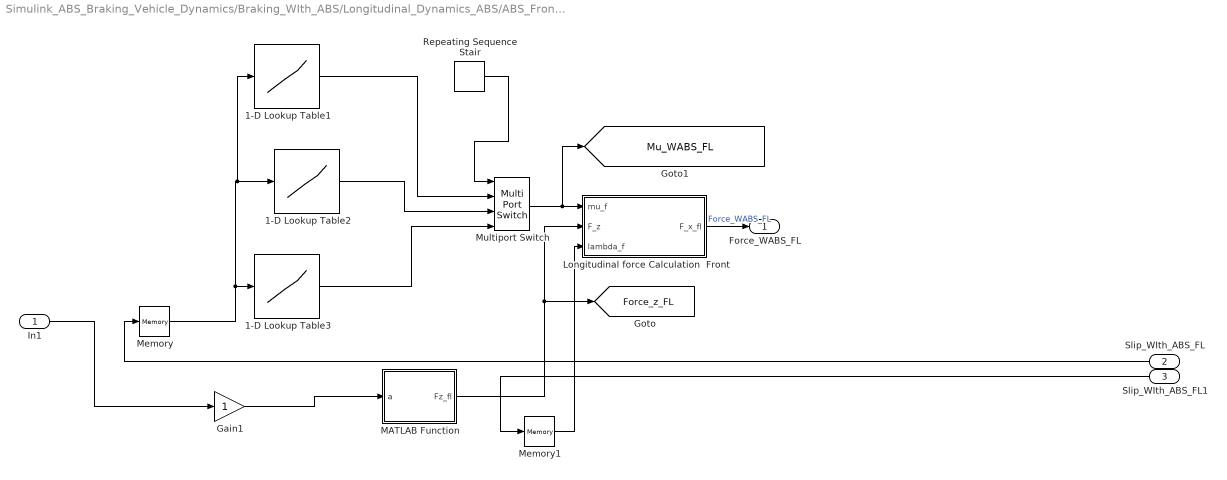
== system Simulink_ABS_Braking_Vehicle_Dynamics/Braking_WIth_ABS/Longitudinal_Dynamics_ABS/ABS_Front_LEFT/Force_Calculation ==
  In1 : Inport
  Slip_WIth_ABS_FL : Inport  Port=2
  Slip_WIth_ABS_FL1 : Inport  Port=3
  1-D Lookup Table1 : Lookup_n-D  NumberOfTableDimensions=1  BreakpointsForDimension1=lambda_bp  Table=mu_dry  InternalRulePriority=Speed  RndMeth=Simplest
  1-D Lookup Table2 : Lookup_n-D  NumberOfTableDimensions=1  BreakpointsForDimension1=lambda_bp  Table=mu_wet  InternalRulePriority=Speed  RndMeth=Simplest
  1-D Lookup Table3 : Lookup_n-D  NumberOfTableDimensions=1  BreakpointsForDimension1=lambda_bp  Table=mu_ice  InternalRulePriority=Speed  RndMeth=Simplest
  Gain1 : Gain
  Longitudinal force Calculation  Front : MATLAB Function  TreatAsAtomicUnit=on
  MATLAB Function : MATLAB Function  TreatAsAtomicUnit=on
  Memory : Memory
  Memory1 : Memory
  Multiport Switch : MultiPortSwitch  SaturateOnIntegerOverflow=off  InputSameDT=off
  Repeating Sequence Stair : simulink/Sources/Repeating Sequence Stair  OutValues=roadSequence  tsamp=time_Road_Sequence  OutMin=[]  OutMax=[]  OutDataTypeStr=double  OutputDataTypeScalingMode=double  OutDataType=fixdt(0,8)  ConRadixGroup=Best Precision: Vector-wise  OutScaling=2^-12
  Force_WABS_FL : Outport
  tag scope: Force_z_FL=global, Mu_WABS_FL=global
  wires:
  MATLAB Function/1(Fz_fl) -> [Force_z_FL], Longitudinal force Calculation  Front/2(F_z)
  Memory/1 -> 1-D Lookup Table3/1, 1-D Lookup Table1/1, 1-D Lookup Table2/1
  Longitudinal force Calculation  Front/1(F_x_fl) -> Force_WABS_FL/1  "Force_WABS_FL"
  In1/1 -> Gain1/1
  Gain1/1 -> MATLAB Function/1(a)
  Memory1/1 -> Longitudinal force Calculation  Front/3(lambda_f)
  Slip_WIth_ABS_FL/1 -> Memory/1
  1-D Lookup Table1/1 -> Multiport Switch/2
  Multiport Switch/1 -> [Mu_WABS_FL], Longitudinal force Calculation  Front/1(mu_f)
  1-D Lookup Table2/1 -> Multiport Switch/3
  Repeating Sequence Stair/1 -> Multiport Switch/1
  1-D Lookup Table3/1 -> Multiport Switch/4
  Slip_WIth_ABS_FL1/1 -> Memory1/1

== system Simulink_ABS_Braking_Vehicle_Dynamics/Braking_WIth_ABS/Longitudinal_Dynamics_ABS/ABS_Front_LEFT/Slip Calculation_ABS ==
  v : Inport
  w : Inport  Port=2
  Constant3 : Constant  Value=r
  MATLAB Function2 : MATLAB Function  TreatAsAtomicUnit=on
  lambda : Outport
  wires:
  w/1 -> MATLAB Function2/3(w)
  MATLAB Function2/1(lambda) -> lambda/1
  v/1 -> MATLAB Function2/1(v)
  Constant3/1 -> MATLAB Function2/2(r)

== system Simulink_ABS_Braking_Vehicle_Dynamics/Braking_WIth_ABS/Longitudinal_Dynamics_ABS/ABS_Front_LEFT/angular_accelration_withABS ==
  F_x : Inport
  usage_FL : Inport  Port=2
  T_brake : Inport  Port=3
  Constant1 : Constant  Value=r
  Constant2 : Constant  Value=I_w
  MATLAB Function : MATLAB Function  TreatAsAtomicUnit=on
  MATLAB Function1 : MATLAB Function  TreatAsAtomicUnit=on
  dw_dt : Outport
  wires:
  Constant2/1 -> MATLAB Function1/4(I_w)
  Constant1/1 -> MATLAB Function1/2(r)
  F_x/1 -> MATLAB Function1/3(F_x_lf)
  MATLAB Function1/1(dw_dt) -> dw_dt/1
  T_brake/1 -> MATLAB Function/1(T_brake_PID)
  usage_FL/1 -> MATLAB Function/2(usage)
  MATLAB Function/1(T_brake_mod) -> MATLAB Function1/1(T_brake)

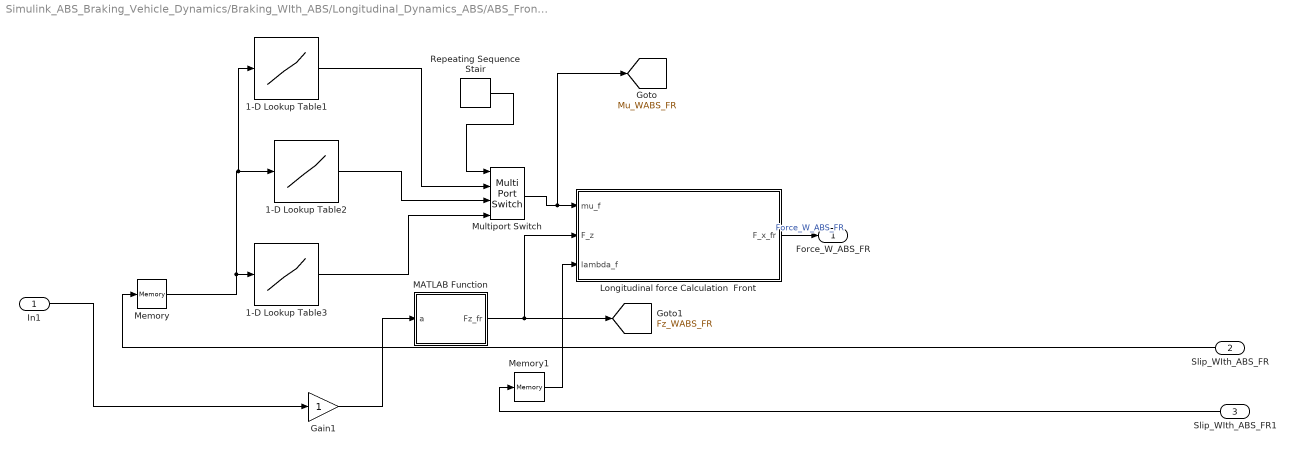
== system Simulink_ABS_Braking_Vehicle_Dynamics/Braking_WIth_ABS/Longitudinal_Dynamics_ABS/ABS_Front_Right/Force_Calculation ==
  In1 : Inport
  Slip_WIth_ABS_FR : Inport  Port=2
  Slip_WIth_ABS_FR1 : Inport  Port=3
  1-D Lookup Table1 : Lookup_n-D  NumberOfTableDimensions=1  BreakpointsForDimension1=lambda_bp  Table=mu_dry  InternalRulePriority=Speed  RndMeth=Simplest
  1-D Lookup Table2 : Lookup_n-D  NumberOfTableDimensions=1  BreakpointsForDimension1=lambda_bp  Table=mu_wet  InternalRulePriority=Speed  RndMeth=Simplest
  1-D Lookup Table3 : Lookup_n-D  NumberOfTableDimensions=1  BreakpointsForDimension1=lambda_bp  Table=mu_ice  InternalRulePriority=Speed  RndMeth=Simplest
  Gain1 : Gain
  Longitudinal force Calculation  Front : MATLAB Function  TreatAsAtomicUnit=on
  MATLAB Function : MATLAB Function  TreatAsAtomicUnit=on
  Memory : Memory
  Memory1 : Memory
  Multiport Switch : MultiPortSwitch  SaturateOnIntegerOverflow=off  InputSameDT=off
  Repeating Sequence Stair : simulink/Sources/Repeating Sequence Stair  OutValues=roadSequence  tsamp=time_Road_Sequence  OutMin=[]  OutMax=[]  OutDataTypeStr=double  OutputDataTypeScalingMode=double  OutDataType=fixdt(0,8)  ConRadixGroup=Best Precision: Vector-wise  OutScaling=2^-12
  Force_W_ABS_FR : Outport
  tag scope: Fz_WABS_FR=global, Mu_WABS_FR=global
  wires:
  In1/1 -> Gain1/1
  Memory/1 -> 1-D Lookup Table2/1, 1-D Lookup Table1/1, 1-D Lookup Table3/1
  1-D Lookup Table2/1 -> Multiport Switch/3
  MATLAB Function/1(Fz_fr) -> Longitudinal force Calculation  Front/2(F_z), [Fz_WABS_FR]
  Repeating Sequence Stair/1 -> Multiport Switch/1
  1-D Lookup Table1/1 -> Multiport Switch/2
  Gain1/1 -> MATLAB Function/1(a)
  1-D Lookup Table3/1 -> Multiport Switch/4
  Longitudinal force Calculation  Front/1(F_x_fr) -> Force_W_ABS_FR/1  "Force_W_ABS_FR"
  Memory1/1 -> Longitudinal force Calculation  Front/3(lambda_f)
  Multiport Switch/1 -> [Mu_WABS_FR], Longitudinal force Calculation  Front/1(mu_f)
  Slip_WIth_ABS_FR1/1 -> Memory1/1
  Slip_WIth_ABS_FR/1 -> Memory/1

== system Simulink_ABS_Braking_Vehicle_Dynamics/Braking_WIth_ABS/Longitudinal_Dynamics_ABS/ABS_Front_Right/Slip Calculation_ABS ==
  v : Inport
  w : Inport  Port=2
  Constant3 : Constant  Value=r
  MATLAB Function2 : MATLAB Function  TreatAsAtomicUnit=on
  lambda : Outport
  wires:
  Constant3/1 -> MATLAB Function2/2(r)
  v/1 -> MATLAB Function2/1(v)
  MATLAB Function2/1(lambda) -> lambda/1
  w/1 -> MATLAB Function2/3(w)

== system Simulink_ABS_Braking_Vehicle_Dynamics/Braking_WIth_ABS/Longitudinal_Dynamics_ABS/ABS_Front_Right/angular_accelration_withABS ==
  F_x_fr : Inport
  usage_FL : Inport  Port=2
  T_brake : Inport  Port=3
  Constant1 : Constant  Value=r
  Constant2 : Constant  Value=I_w
  MATLAB Function : MATLAB Function  TreatAsAtomicUnit=on
  MATLAB Function1 : MATLAB Function  TreatAsAtomicUnit=on
  dw_dt : Outport
  wires:
  MATLAB Function1/1(dw_dt) -> dw_dt/1
  F_x_fr/1 -> MATLAB Function1/3(F_x_fr)
  Constant1/1 -> MATLAB Function1/2(r)
  Constant2/1 -> MATLAB Function1/4(I_w)
  T_brake/1 -> MATLAB Function/1(T_brake_PID)
  usage_FL/1 -> MATLAB Function/2(usage)
  MATLAB Function/1(T_brake_mod) -> MATLAB Function1/1(T_brake)

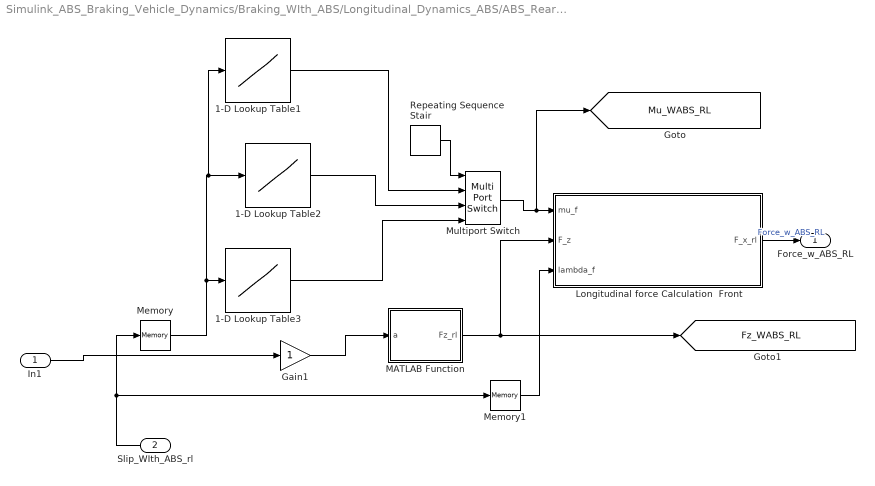
== system Simulink_ABS_Braking_Vehicle_Dynamics/Braking_WIth_ABS/Longitudinal_Dynamics_ABS/ABS_Rear_Left/Force_Caculation ==
  In1 : Inport
  Slip_WIth_ABS_rl : Inport  Port=2
  1-D Lookup Table1 : Lookup_n-D  NumberOfTableDimensions=1  BreakpointsForDimension1=lambda_bp  Table=mu_dry  InternalRulePriority=Speed  RndMeth=Simplest
  1-D Lookup Table2 : Lookup_n-D  NumberOfTableDimensions=1  BreakpointsForDimension1=lambda_bp  Table=mu_wet  InternalRulePriority=Speed  RndMeth=Simplest
  1-D Lookup Table3 : Lookup_n-D  NumberOfTableDimensions=1  BreakpointsForDimension1=lambda_bp  Table=mu_ice  InternalRulePriority=Speed  RndMeth=Simplest
  Gain1 : Gain
  Longitudinal force Calculation  Front : MATLAB Function  TreatAsAtomicUnit=on
  MATLAB Function : MATLAB Function  TreatAsAtomicUnit=on
  Memory : Memory
  Memory1 : Memory
  Multiport Switch : MultiPortSwitch  SaturateOnIntegerOverflow=off  InputSameDT=off
  Repeating Sequence Stair : simulink/Sources/Repeating Sequence Stair  OutValues=roadSequence  tsamp=time_Road_Sequence  OutMin=[]  OutMax=[]  OutDataTypeStr=double  OutputDataTypeScalingMode=double  OutDataType=fixdt(0,8)  ConRadixGroup=Best Precision: Vector-wise  OutScaling=2^-12
  Force_w_ABS_RL : Outport
  tag scope: Fz_WABS_RL=global, Mu_WABS_RL=global
  wires:
  In1/1 -> Gain1/1
  Memory/1 -> 1-D Lookup Table3/1, 1-D Lookup Table1/1, 1-D Lookup Table2/1
  Longitudinal force Calculation  Front/1(F_x_rl) -> Force_w_ABS_RL/1  "Force_w_ABS_RL"
  Slip_WIth_ABS_rl/1 -> Memory/1, Memory1/1
  Gain1/1 -> MATLAB Function/1(a)
  1-D Lookup Table3/1 -> Multiport Switch/4
  Repeating Sequence Stair/1 -> Multiport Switch/1
  MATLAB Function/1(Fz_rl) -> Longitudinal force Calculation  Front/2(F_z), [Fz_WABS_RL]
  Multiport Switch/1 -> [Mu_WABS_RL], Longitudinal force Calculation  Front/1(mu_f)
  1-D Lookup Table1/1 -> Multiport Switch/2
  Memory1/1 -> Longitudinal force Calculation  Front/3(lambda_f)
  1-D Lookup Table2/1 -> Multiport Switch/3

== system Simulink_ABS_Braking_Vehicle_Dynamics/Braking_WIth_ABS/Longitudinal_Dynamics_ABS/ABS_Rear_Left/Slip Calculation_ABS_rl ==
  v : Inport
  w : Inport  Port=2
  Constant3 : Constant  Value=r
  MATLAB Function2 : MATLAB Function  TreatAsAtomicUnit=on
  lambda : Outport
  wires:
  w/1 -> MATLAB Function2/3(w)
  MATLAB Function2/1(lambda) -> lambda/1
  v/1 -> MATLAB Function2/1(v)
  Constant3/1 -> MATLAB Function2/2(r)

== system Simulink_ABS_Braking_Vehicle_Dynamics/Braking_WIth_ABS/Longitudinal_Dynamics_ABS/ABS_Rear_Left/angular_accelration_withABS ==
  F_x_rl : Inport
  usage_FL : Inport  Port=2
  T_brake : Inport  Port=3
  Constant1 : Constant  Value=r
  Constant2 : Constant  Value=I_w
  MATLAB Function : MATLAB Function  TreatAsAtomicUnit=on
  MATLAB Function1 : MATLAB Function  TreatAsAtomicUnit=on
  dw_dt : Outport
  wires:
  Constant2/1 -> MATLAB Function1/4(I_w)
  Constant1/1 -> MATLAB Function1/2(r)
  F_x_rl/1 -> MATLAB Function1/3(F_x_rl)
  MATLAB Function1/1(dw_dt) -> dw_dt/1
  T_brake/1 -> MATLAB Function/1(T_brake_PID)
  usage_FL/1 -> MATLAB Function/2(usage)
  MATLAB Function/1(T_brake_mod) -> MATLAB Function1/1(T_brake)

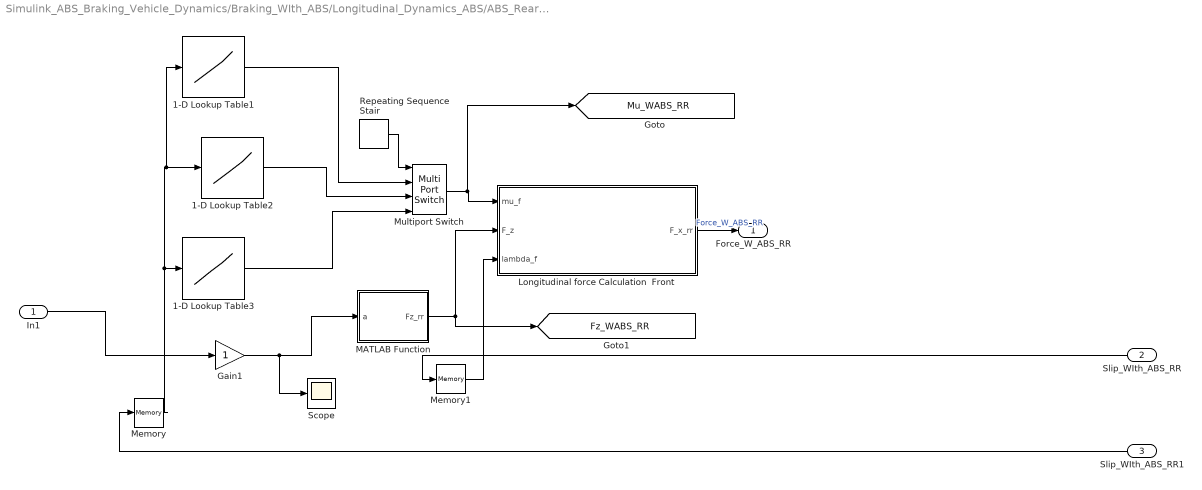
== system Simulink_ABS_Braking_Vehicle_Dynamics/Braking_WIth_ABS/Longitudinal_Dynamics_ABS/ABS_Rear_Right/Force_Calculation_Rear_Right ==
  In1 : Inport
  Slip_WIth_ABS_RR : Inport  Port=2
  Slip_WIth_ABS_RR1 : Inport  Port=3
  1-D Lookup Table1 : Lookup_n-D  NumberOfTableDimensions=1  BreakpointsForDimension1=lambda_bp  Table=mu_dry  InternalRulePriority=Speed  RndMeth=Simplest
  1-D Lookup Table2 : Lookup_n-D  NumberOfTableDimensions=1  BreakpointsForDimension1=lambda_bp  Table=mu_wet  InternalRulePriority=Speed  RndMeth=Simplest
  1-D Lookup Table3 : Lookup_n-D  NumberOfTableDimensions=1  BreakpointsForDimension1=lambda_bp  Table=mu_ice  InternalRulePriority=Speed  RndMeth=Simplest
  Gain1 : Gain
  Longitudinal force Calculation  Front : MATLAB Function  TreatAsAtomicUnit=on
  MATLAB Function : MATLAB Function  TreatAsAtomicUnit=on
  Memory : Memory
  Memory1 : Memory
  Multiport Switch : MultiPortSwitch  SaturateOnIntegerOverflow=off  InputSameDT=off
  Repeating Sequence Stair : simulink/Sources/Repeating Sequence Stair  OutValues=roadSequence  tsamp=time_Road_Sequence  OutMin=[]  OutMax=[]  OutDataTypeStr=double  OutputDataTypeScalingMode=double  OutDataType=fixdt(0,8)  ConRadixGroup=Best Precision: Vector-wise  OutScaling=2^-12
  Scope : Scope
  Force_W_ABS_RR : Outport
  tag scope: Fz_WABS_RR=global, Mu_WABS_RR=global
  wires:
  Longitudinal force Calculation  Front/1(F_x_rr) -> Force_W_ABS_RR/1  "Force_W_ABS_RR"
  Memory/1 -> 1-D Lookup Table2/1, 1-D Lookup Table1/1, 1-D Lookup Table3/1
  1-D Lookup Table2/1 -> Multiport Switch/3
  MATLAB Function/1(Fz_rr) -> Longitudinal force Calculation  Front/2(F_z), [Fz_WABS_RR]
  Repeating Sequence Stair/1 -> Multiport Switch/1
  1-D Lookup Table1/1 -> Multiport Switch/2
  Multiport Switch/1 -> [Mu_WABS_RR], Longitudinal force Calculation  Front/1(mu_f)
  Memory1/1 -> Longitudinal force Calculation  Front/3(lambda_f)
  Gain1/1 -> Scope/1, MATLAB Function/1(a)
  1-D Lookup Table3/1 -> Multiport Switch/4
  In1/1 -> Gain1/1
  Slip_WIth_ABS_RR/1 -> Memory1/1
  Slip_WIth_ABS_RR1/1 -> Memory/1

== system Simulink_ABS_Braking_Vehicle_Dynamics/Braking_WIth_ABS/Longitudinal_Dynamics_ABS/ABS_Rear_Right/Slip Calculation_ABS_rl ==
  v : Inport
  w : Inport  Port=2
  Constant3 : Constant  Value=r
  MATLAB Function2 : MATLAB Function  TreatAsAtomicUnit=on
  lambda : Outport
  wires:
  Constant3/1 -> MATLAB Function2/2(r)
  v/1 -> MATLAB Function2/1(v)
  MATLAB Function2/1(lambda) -> lambda/1
  w/1 -> MATLAB Function2/3(w)

== system Simulink_ABS_Braking_Vehicle_Dynamics/Braking_WIth_ABS/Longitudinal_Dynamics_ABS/ABS_Rear_Right/angular_accelration_withABS ==
  F_x_rr : Inport
  usage_FL : Inport  Port=2
  T_brake : Inport  Port=3
  Constant1 : Constant  Value=r
  Constant2 : Constant  Value=I_w
  MATLAB Function : MATLAB Function  TreatAsAtomicUnit=on
  MATLAB Function1 : MATLAB Function  TreatAsAtomicUnit=on
  dw_dt : Outport
  wires:
  MATLAB Function1/1(dw_dt) -> dw_dt/1
  F_x_rr/1 -> MATLAB Function1/3(F_x_rr)
  Constant1/1 -> MATLAB Function1/2(r)
  Constant2/1 -> MATLAB Function1/4(I_w)
  T_brake/1 -> MATLAB Function/1(T_brake_PID)
  MATLAB Function/1(T_brake_mod) -> MATLAB Function1/1(T_brake)
  usage_FL/1 -> MATLAB Function/2(usage)

== system Simulink_ABS_Braking_Vehicle_Dynamics/Braking_Without_ABS/Longitudinal_dynamics/Front_Wheel_left_CAlculation/Slip Calculation ==
  v : Inport
  w : Inport  Port=2
  Constant3 : Constant  Value=r
  MATLAB Function2 : MATLAB Function  TreatAsAtomicUnit=on
  lambda : Outport
  wires:
  Constant3/1 -> MATLAB Function2/2(r)
  v/1 -> MATLAB Function2/1(v)
  MATLAB Function2/1(lambda) -> lambda/1
  w/1 -> MATLAB Function2/3(w_lf)

== system Simulink_ABS_Braking_Vehicle_Dynamics/Braking_Without_ABS/Longitudinal_dynamics/Front_Wheel_left_CAlculation/Vehicle Speed_Block ==
  a : Inport
  Constant3 : Constant  Value=0.8
  Constant4 : Constant  Value=0.55
  Constant5 : Constant  Value=0.14
  Force_Calculation_No_ABS : MATLAB Function  TreatAsAtomicUnit=on
  MATLAB Function : MATLAB Function  TreatAsAtomicUnit=on
  Multiport Switch : MultiPortSwitch  SaturateOnIntegerOverflow=off  InputSameDT=off
  Repeating Sequence Stair : simulink/Sources/Repeating Sequence Stair  OutValues=roadSequence  tsamp=time_Road_Sequence  OutMin=[]  OutMax=[]  OutDataTypeStr=double  OutputDataTypeScalingMode=double  OutDataType=fixdt(0,8)  ConRadixGroup=Best Precision: Vector-wise  OutScaling=2^-12
  F_x : Outport
  wires:
  Force_Calculation_No_ABS/1(F_x_fl) -> F_x/1
  MATLAB Function/1(Fz_fl) -> Force_Calculation_No_ABS/2(F_z)
  Constant5/1 -> Multiport Switch/4
  Constant3/1 -> Multiport Switch/2
  Constant4/1 -> Multiport Switch/3
  Repeating Sequence Stair/1 -> Multiport Switch/1
  Multiport Switch/1 -> Force_Calculation_No_ABS/1(mu)
  a/1 -> MATLAB Function/1(a)

== system Simulink_ABS_Braking_Vehicle_Dynamics/Braking_Without_ABS/Longitudinal_dynamics/Front_Wheel_left_CAlculation/angular_accelration_Wo_ABS ==
  F_xf : Inport
  Constant : Constant  Value=T_brake
  Constant1 : Constant  Value=r
  Constant2 : Constant  Value=I_w
  MATLAB Function1 : MATLAB Function  TreatAsAtomicUnit=on
  dw_dt : Outport
  wires:
  Constant1/1 -> MATLAB Function1/2(r)
  Constant2/1 -> MATLAB Function1/4(I_w)
  MATLAB Function1/1(dw_dt) -> dw_dt/1
  F_xf/1 -> MATLAB Function1/3(F_x_lf)
  Constant/1 -> MATLAB Function1/1(T_brake)

== system Simulink_ABS_Braking_Vehicle_Dynamics/Braking_Without_ABS/Longitudinal_dynamics/Front_Wheel_right_CAlculation/Slip Calculation ==
  v : Inport
  w : Inport  Port=2
  Constant3 : Constant  Value=r
  MATLAB Function2 : MATLAB Function  TreatAsAtomicUnit=on
  lambda : Outport
  wires:
  Constant3/1 -> MATLAB Function2/2(r)
  v/1 -> MATLAB Function2/1(v)
  MATLAB Function2/1(lambda) -> lambda/1
  w/1 -> MATLAB Function2/3(w)

== system Simulink_ABS_Braking_Vehicle_Dynamics/Braking_Without_ABS/Longitudinal_dynamics/Front_Wheel_right_CAlculation/Vehicle Speed_Block ==
  a : Inport
  Constant3 : Constant  Value=0.8
  Constant4 : Constant  Value=0.55
  Constant5 : Constant  Value=0.14
  Force_Calculation_No_ABS : MATLAB Function  TreatAsAtomicUnit=on
  MATLAB Function : MATLAB Function  TreatAsAtomicUnit=on
  Multiport Switch : MultiPortSwitch  SaturateOnIntegerOverflow=off  InputSameDT=off
  Repeating Sequence Stair : simulink/Sources/Repeating Sequence Stair  OutValues=roadSequence  tsamp=time_Road_Sequence  OutMin=[]  OutMax=[]  OutDataTypeStr=double  OutputDataTypeScalingMode=double  OutDataType=fixdt(0,8)  ConRadixGroup=Best Precision: Vector-wise  OutScaling=2^-12
  F_x_fr : Outport
  wires:
  Force_Calculation_No_ABS/1(F_x_fr) -> F_x_fr/1
  Constant5/1 -> Multiport Switch/4
  Constant3/1 -> Multiport Switch/2
  Constant4/1 -> Multiport Switch/3
  Repeating Sequence Stair/1 -> Multiport Switch/1
  Multiport Switch/1 -> Force_Calculation_No_ABS/1(mu)
  MATLAB Function/1(Fz_fr) -> Force_Calculation_No_ABS/2(F_z)
  a/1 -> MATLAB Function/1(a)

== system Simulink_ABS_Braking_Vehicle_Dynamics/Braking_Without_ABS/Longitudinal_dynamics/Front_Wheel_right_CAlculation/angular_accelration_Wo_ABS ==
  F_x_fr : Inport
  Constant : Constant  Value=T_brake
  Constant1 : Constant  Value=r
  Constant2 : Constant  Value=I_w
  MATLAB Function1 : MATLAB Function  TreatAsAtomicUnit=on
  dw_dt : Outport
  wires:
  Constant1/1 -> MATLAB Function1/2(r)
  Constant2/1 -> MATLAB Function1/4(I_w)
  MATLAB Function1/1(dw_dt) -> dw_dt/1
  F_x_fr/1 -> MATLAB Function1/3(F_x_fr)
  Constant/1 -> MATLAB Function1/1(T_brake)

== system Simulink_ABS_Braking_Vehicle_Dynamics/Braking_Without_ABS/Longitudinal_dynamics/Rear_Wheel_Right_CAlculation/Slip Calculation ==
  v : Inport
  w : Inport  Port=2
  Constant3 : Constant  Value=r
  MATLAB Function2 : MATLAB Function  TreatAsAtomicUnit=on
  lambda : Outport
  wires:
  w/1 -> MATLAB Function2/3(w)
  MATLAB Function2/1(lambda) -> lambda/1
  v/1 -> MATLAB Function2/1(v)
  Constant3/1 -> MATLAB Function2/2(r)

== system Simulink_ABS_Braking_Vehicle_Dynamics/Braking_Without_ABS/Longitudinal_dynamics/Rear_Wheel_Right_CAlculation/Vehicle Speed_Block ==
  a : Inport
  Constant3 : Constant  Value=0.8
  Constant4 : Constant  Value=0.55
  Constant5 : Constant  Value=0.14
  Force_Calculation_No_ABS : MATLAB Function  TreatAsAtomicUnit=on
  MATLAB Function : MATLAB Function  TreatAsAtomicUnit=on
  Multiport Switch : MultiPortSwitch  SaturateOnIntegerOverflow=off  InputSameDT=off
  Repeating Sequence Stair : simulink/Sources/Repeating Sequence Stair  OutValues=roadSequence  tsamp=time_Road_Sequence  OutMin=[]  OutMax=[]  OutDataTypeStr=double  OutputDataTypeScalingMode=double  OutDataType=fixdt(0,8)  ConRadixGroup=Best Precision: Vector-wise  OutScaling=2^-12
  F_x_RR : Outport
  wires:
  Multiport Switch/1 -> Force_Calculation_No_ABS/1(mu)
  Repeating Sequence Stair/1 -> Multiport Switch/1
  Constant4/1 -> Multiport Switch/3
  Constant3/1 -> Multiport Switch/2
  Constant5/1 -> Multiport Switch/4
  Force_Calculation_No_ABS/1(F_x_RR) -> F_x_RR/1
  MATLAB Function/1(Fz_rr) -> Force_Calculation_No_ABS/2(F_z)
  a/1 -> MATLAB Function/1(a)
